simulink model "explicitaccel"  (R2021a)
settings: Solver=FixedStepAuto  StartTime=0.0  StopTime=inf  FixedStep=0.1  RelTol=1e-3
undefined symbols (not defined in the file): Angular, Linear
libraries: robotlib x20
settings Model: Creator=ivory  LastModifiedBy=sprinkle
settings SolverCC: AlgebraicLoopSolver=TrustRegion
settings OptimizationCC: EnhancedBackFolding=on  PassReuseOutputArgsAs=Individual arguments  ZeroExternalMemoryAtStartup=off  ZeroInternalMemoryAtStartup=off  MaxStackSize=64  OptimizeBlockOrder=speed  DifferentSizesBufferReuse=on  OptimizationCustomize=off  EfficientTunableParamExpr=on
settings DebuggingCC: ParameterTunabilityLossMsg=error  SFMachineParentedDataDiag=warning
settings HardwareCC: ProdBitPerPointer=32  ProdBitPerSizeT=32  ProdBitPerPtrDiffT=32  ProdLargestAtomicFloat=None  ProdIntDivRoundTo=Undefined  ProdEndianess=Unspecified  ProdWordSize=32  ProdHWDeviceType=Generic->Unspecified (assume 32-bit Generic)
settings SFSimCC: MATLABDynamicMemAlloc=off  SimTargetLang=C++
settings RTWCC: SystemTargetFile=ert.tlc  HardwareBoard=Robot Operating System (ROS)  TLCOptions="-aInlineSetEventsForThisBaseRateFcn=TLC_FALSE -aSuppressMultiTaskScheduler=TLC_FALSE  -aRateBasedStepFcn=0"  TemplateMakefile=ert_default_tmf  GenerateReport=on  Toolchain=Catkin  IncludeHyperlinkInReport=on  LaunchReport=on  TargetLang=C++  GenerateTraceInfo=on  GenerateTraceReport=on  GenerateTraceReportSl=on  GenerateTraceReportSf=on  GenerateTraceReportEml=on
settings CodeAppCC: ForceParamTrailComments=on  IgnoreCustomStorageClasses=off  OperatorAnnotations=on  SimulinkDataObjDesc=on  SFDataObjDesc=on  InsertBlockDesc=on
settings ERTTargetCC: SupportContinuousTime=on  SupportVariableSizeSignals=on

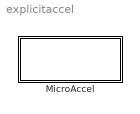
== system explicitaccel ==
  MicroAccel : Subsystem

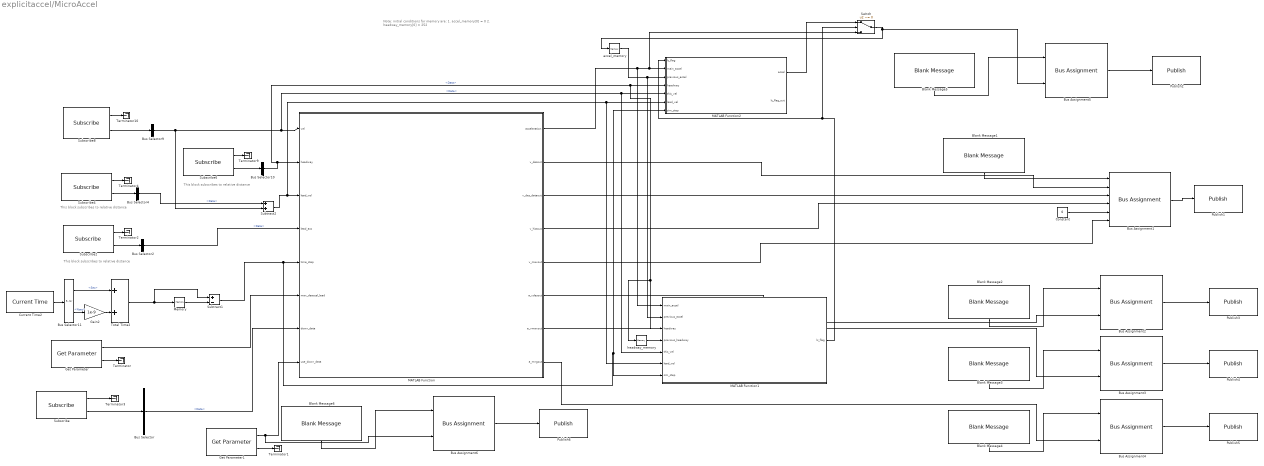
== system explicitaccel/MicroAccel ==
  note: Note: initial conditions for memory are:
      |
      | 1. accel_memory[0] = 0
      | 2. headway_memory[0] = 252
  note: This block subscribes
      | to relative distance
  note: This block subscribes
      | to relative distance
  note: This block subscribes
      | to relative distance
  Blank Message1 : robotlib/Blank Message  messageClass=Message  entityType=geometry_msgs/Twist  messageType=geometry_msgs/Twist  SampleTime=inf  legacyBusStruct=off
  Blank Message{2..5} (4 alike) : robotlib/Blank Message  messageClass=Message  entityType=std_msgs/Float64  messageType=std_msgs/Float64  SampleTime=inf  legacyBusStruct=off
  Blank Message6 : robotlib/Blank Message  messageClass=Message  entityType=std_msgs/Bool  messageType=std_msgs/Bool  SampleTime=inf  legacyBusStruct=off
  Bus Assignment1 : BusAssignment  AssignedSignals=Linear.X,Linear.Y,Linear.Z,Angular.Z,Angular.X
  Bus Assignment{2..6} (5 alike) : BusAssignment  AssignedSignals=Data
  Bus Selector{,2,4,9..10} (5 alike) : BusSelector  OutputSignals=Data
  Bus Selector11 : BusSelector  OutputSignals=Sec,Nsec
  Constant : Constant  Value=0
  Current Time2 : robotlib/Current Time  OutputFormat=bus  SampleTime=-1  ModelName=explicitaccel
      settings: SourceProductBaseCode=RR
  Gain2 : Gain  Gain=1e-9
  Get Parameter : robotlib/Get Parameter  ParameterSource=Specify your own  ParameterName=max_deaccel_lead  ParameterType=double  ParameterMaxArrayLength=16  ParameterInitialValue=-4.5  SampleTime=-1  ShowErrorCodeOutput=on  ModelName=explicitaccel  BlockId=ParamGet_explicitaccel_585
      settings: SourceProductBaseCode=RR
  Get Parameter1 : robotlib/Get Parameter  ParameterSource=Specify your own  ParameterName=use_down_data  ParameterType=boolean  ParameterMaxArrayLength=16  ParameterInitialValue=0.0  SampleTime=-1  ShowErrorCodeOutput=on  ModelName=explicitaccel  BlockId=ParamGet_explicitaccel_631
      settings: SourceProductBaseCode=RR
  MATLAB Function : MATLAB Function  TreatAsAtomicUnit=on
  MATLAB Function1 : MATLAB Function  TreatAsAtomicUnit=on
  MATLAB Function2 : MATLAB Function  TreatAsAtomicUnit=on
  Memory : Memory
  Publish1 : robotlib/Publish  topicSource=Specify your own  topic=cmd_vel  messageType=geometry_msgs/Twist  legacyBusStruct=off  messageQueueLength=1
  Publish2 : robotlib/Publish  topicSource=Specify your own  topic=cmd_accel  messageType=std_msgs/Float64  legacyBusStruct=off  messageQueueLength=1
  Publish3 : robotlib/Publish  topicSource=Specify your own  topic=a_vdesout  messageType=std_msgs/Float64  legacyBusStruct=off  messageQueueLength=1
  Publish4 : robotlib/Publish  topicSource=Specify your own  topic=a_vmaxout  messageType=std_msgs/Float64  legacyBusStruct=off  messageQueueLength=1
  Publish5 : robotlib/Publish  topicSource=Specify your own  topic=a_mngout  messageType=std_msgs/Float64  legacyBusStruct=off  messageQueueLength=1
  Publish6 : robotlib/Publish  topicSource=Specify your own  topic=downdataflag  messageType=std_msgs/Bool  legacyBusStruct=off  messageQueueLength=1
  Subscribe : robotlib/Subscribe  topicSource=Specify your own  topic=down_data  messageType=std_msgs/Float64MultiArray  SampleTime=-1  legacyBusStruct=off  messageQueueLength=1
  Subscribe2 : robotlib/Subscribe  topicSource=Specify your own  topic=lead_accel  messageType=std_msgs/Float64  SampleTime=-1  legacyBusStruct=off  messageQueueLength=1
  Subscribe4 : robotlib/Subscribe  topicSource=Specify your own  topic=rel_vel  messageType=std_msgs/Float64  SampleTime=-1  legacyBusStruct=off  messageQueueLength=1
  Subscribe6 : robotlib/Subscribe  topicSource=Specify your own  topic=lead_dist  messageType=std_msgs/Float64  SampleTime=-1  legacyBusStruct=off  messageQueueLength=1
  Subscribe8 : robotlib/Subscribe  topicSource=Specify your own  topic=vel  messageType=std_msgs/Float64  SampleTime=-1  legacyBusStruct=off  messageQueueLength=1
  Subtract1 : Sum  Inputs=+-
  Subtract2 : Sum
  Switch : Switch  Criteria=u2 ~= 0
  Terminator{,1..4,9..10} (7 alike) : Terminator
  Total Time2 : Sum
  accel_memory : Memory
  headway_memory : Memory  InitialCondition=252
  wires:
  Subscribe8/1 -> Terminator10/1
  Subscribe8/2 -> Bus Selector9/1
  Bus Selector9/1 -> MATLAB Function1/5(this_vel), MATLAB Function2/5(this_vel), MATLAB Function/1(vel), Subtract2/2  "<Data>"
  Subscribe6/1 -> Terminator9/1
  Subscribe6/2 -> Bus Selector10/1
  Bus Selector10/1 -> MATLAB Function/2(headway), headway_memory/1, MATLAB Function1/3(headway), MATLAB Function2/4(headway)  "<Data>"
  Bus Selector2/1 -> MATLAB Function/4(lead_acc)  "<Data>"
  Subscribe2/2 -> Bus Selector2/1
  Subscribe2/1 -> Terminator2/1
  Bus Selector11/1 -> Total Time2/1  "<Sec>"
  Gain2/1 -> Total Time2/2
  Bus Selector11/2 -> Gain2/1  "<Nsec>"
  Total Time2/1 -> Subtract1/1, Memory/1
  Current Time2/1 -> Bus Selector11/1
  Memory/1 -> Subtract1/2
  Subtract1/1 -> MATLAB Function2/7(sim_step), MATLAB Function1/7(sim_step), MATLAB Function/5(time_step)
  Get Parameter/2 -> Terminator/1
  Get Parameter/1 -> MATLAB Function/6(max_deaccel_lead)
  Constant/1 -> Bus Assignment1/5
  Bus Assignment1/1 -> Publish1/1
  MATLAB Function/4(v_histout) -> Bus Assignment1/4
  Blank Message1/1 -> Bus Assignment1/1
  MATLAB Function/3(v_des_dataout) -> Bus Assignment1/3
  MATLAB Function/5(v_maxout) -> Bus Assignment1/6
  MATLAB Function/7(a_vmaxout) -> Bus Assignment3/2
  MATLAB Function/2(v_desout) -> Bus Assignment1/2
  Subscribe/1 -> Terminator3/1
  Subscribe/2 -> Bus Selector/1
  Bus Selector/1 -> MATLAB Function/7(down_data)  "<Data>"
  Blank Message2/1 -> Bus Assignment2/1
  MATLAB Function/6(a_vdesout) -> Bus Assignment2/2
  Blank Message3/1 -> Bus Assignment3/1
  Blank Message4/1 -> Bus Assignment4/1
  Blank Message5/1 -> Bus Assignment5/1
  MATLAB Function/1(acceleration) -> MATLAB Function1/1(main_accel), Switch/3, MATLAB Function2/2(main_accel)
  Bus Assignment5/1 -> Publish2/1
  Bus Assignment2/1 -> Publish3/1
  Bus Assignment3/1 -> Publish4/1
  Bus Assignment4/1 -> Publish5/1
  MATLAB Function/8(a_mngout) -> Bus Assignment4/2
  Bus Selector4/1 -> Subtract2/1  "<Data>"
  Subscribe4/2 -> Bus Selector4/1
  Subscribe4/1 -> Terminator4/1
  Subtract2/1 -> MATLAB Function1/6(lead_vel), MATLAB Function2/6(lead_vel), MATLAB Function/3(lead_vel)
  Get Parameter1/2 -> Terminator1/1
  Bus Assignment6/1 -> Publish6/1
  Get Parameter1/1 -> Bus Assignment6/2, MATLAB Function/8(use_down_data)
  Blank Message6/1 -> Bus Assignment6/1
  MATLAB Function1/1(lc_flag) -> Switch/2, MATLAB Function2/1(lc_flag)
  accel_memory/1 -> MATLAB Function1/2(previous_accel), MATLAB Function2/3(previous_accel)
  headway_memory/1 -> MATLAB Function1/4(previous_headway)
  MATLAB Function2/1(accel) -> Switch/1
  Switch/1 -> Bus Assignment5/2, accel_memory/1

== matlab function explicitaccel/MicroAccel/MATLAB Function1 ==
  data: main_accel input; lc_flag output; previous_accel input; headway input; previous_headway input; this_vel input; lead_vel input; sim_step input
function lc_flag = detect_lane_change(main_accel, previous_accel, headway, previous_headway, this_vel, lead_vel, sim_step)
    lc_thresh = 3.5;
    a_comfort = 0.9 * sim_step;
    th_safe = 2;
    ttc_safe = 4.5;

    rv = lead_vel - this_vel;
    da = abs(main_accel - previous_accel);
    
    th = (this_vel > 0) * (headway / this_vel) + (this_vel <= 0) * 60;
    ttc = (rv < 0) * (-headway / rv) +  (rv >= 0) *  60;
    difference = headway - previous_headway;

    if difference <= -lc_thresh
        if da > a_comfort
            if rv >= 0 && th > th_safe
                lc_flag = -1;
                return
            elseif rv < 0 && ttc > ttc_safe
                lc_flag = -1;
                return
            end 
        end 
    elseif difference >= lc_thresh
        if da > a_comfort
            if rv >= 0 && th > th_safe
                lc_flag = 1; 
                return
            elseif rv < 0 && ttc > ttc_safe
                lc_flag = 1; 
                return
            end 
        end
    end 

    lc_flag = 0; 
end

== matlab function explicitaccel/MicroAccel/MATLAB Function ==
  data: vel input; acceleration output; headway input; lead_vel input; lead_acc input; time_step input; max_deaccel_lead input; down_data input; v_desout output; v_des_dataout output; v_histout output; v_maxout output; a_vdesout output; a_vmaxout output; a_mngout output; use_down_data input
function [acceleration, v_desout, v_des_dataout,v_histout, v_maxout, a_vdesout, a_vmaxout, a_mngout]  = Microaccel_05_22(vel, headway, lead_vel, lead_acc, time_step, max_deaccel_lead, down_data, use_down_data)
    %% Compute the desired acceleration by the Microaccel controller.
    % This model requires memory from previous time steps to properly function.
    % To achieve this, we pass the variables to be stored in memory as inputs
    % to the function, and return the updated values as outputs from it. These
    % parameters should be initialized as follows:
    % >>> time_avg_target = [];
    %
    % Parameters
    % ----------
    % vel : float
    %     the speed of the ego vehicle
    % headway : float
    %     bumper-to-bumper gap
    % lead_vel : float
    %     speed of vehicle in front
    % lead_vel : float
    %     accel of vehicle in front
    % time_step : float
    %     the average time (in seconds) in between consecutive updates
    % max_deaccel_lead : float
    %       maximal decceleration achievable by the lead vehicle
    % time_avg_target : list of float
    %     a buffer of leader speeds at previous time steps
    %
    % Returns
    % -------
    % (float, float, float, float, list of float)
    %     the desired acceleration and updated d1, d2, v_des2, and 
    %     time_avg_target terms
    %% model parameters
    max_accel = 1; %Max acceleration
    max_deaccel = -3; %Max decceleration (safety wise)
    max_deaccel_confort = -1; %Max confortable decceleration (i.e. not for safety)
    v_fast = 15;
    v_limit = 30;
    v_hist = 6;
    % to be optimized
    period = 64; 
    weight_des = 1; %parameter always equal to 1 in python, 0 means the have no gap penalty and we don't care about leader vel for v_des
    weight_hist = 0;
    weight_down = 4;
    target_time_head = 3;
    long_time_head = 5;
    h0=2.5;
    s0=2;
    k = 1; %TODO maybe decrease this parameter sometimes
    %options on the controller
    gap_variant = 1; %1 includes a gap preference for the AV, 0 only takes an average
    historical = 0; %0 assumes no past measurments on the test site, 1 uses the data from the known behavior of the traffic without AV
    
    %% Use as input
    %use_down_data = 1; %1 assures to use the downstream information, 0 is to ignore downstream data

    %% Persistent variables
    persistent previous_v_max  %the max velocity for safety in last step
    persistent previous_v_des  %the desired velocity in last step
    persistent previous_dx     %the headway in last step
    persistent time_avg_target %in order to calculate the desried velocity, time_avg_target is the column to memorize the history data
    persistent t_length        %
    average_step = 1280;%period/time_step; %the total number of memory steps
    if isempty(time_avg_target)
        t_length= 1;
        time_avg_target = zeros(1, average_step);% Data Rate = 20 Hz, To consider 64 seconds, 20*64 data points are required
        time_avg_target(average_step)= lead_vel;
    else
        time_avg_target = [time_avg_target(2:end),lead_vel];
        if(t_length < average_step)
            t_length= t_length + 1;
        end
    end
    %% Choose the desired speed based.
    % Create reference values for global target speed.
    % time_avg_target(end+1) = lead_vel
    dx = headway;
    if isempty(previous_dx)
        previous_dx = dx;
    end
    h1= target_time_head.*vel; %%%%here the target time headway is chosen as 3
    %%%%%%%%% Takes care of dowstream_data. Warning: downstream data kind
    %%%%%%%%% of overrides the headway penalization in earlier versions
    if use_down_data == 1 
        v_des_data = min(down_data); %%%%%%%%%down_data is the imported data
    else
        weight_down = 0;
        v_des_data = v_fast;
    end
    if historical == 0
        weight_hist=0;
    end
    v_des = sum(time_avg_target)/t_length; %the desired velocity from the leading vehicle
    if gap_variant == 1 %this parameter is called pen_th in python
       sum_weights = (weight_down + weight_hist + weight_des);
       v_des = (0.1.*max(0,5.*(dx-h1)./max(1, vel))^2+ v_des); %%%%%%%%%Penalise too large headway, the constants can be modified
    end
    v_des = (weight_down * v_des_data + weight_hist * v_hist + weight_des * v_des) / sum_weights; %%%%%%%%%%%%%The desired velocity based on leadign vehicle and downstream info
    %end
    
    
    if isempty(previous_v_des) 
        previous_v_des = 0;
        v_des_dot = 0;
    else
        v_des_dot = (v_des-previous_v_des)./time_step;
    end
    
    previous_v_des = v_des; %update previous_v_des
    % % Compute v_max and its derivative 
    
    v_max = sqrt(2*abs(max_deaccel)*(max(dx-s0,0)+0.5.*((lead_vel).^2)./abs(max_deaccel_lead)));
    if isempty(previous_v_max)
        previous_v_max = 0;
        v_max_dot = 0;
    elseif abs(dx-previous_dx)>time_step * 50 %Exclude the discontinuities in headway 
        v_max_dot = 0;
    else
        v_max_dot = (v_max-previous_v_max)./time_step;
    end
    
    previous_v_max = v_max; %update previous_v_max
    
    %Compute a_mng (acceleration management)
    %%%%%%%%%% Corrected
   
    a_12 = -0.5.*(vel)^2./(max(0,dx-s0)+0.5.*((lead_vel+0.001).^2)./abs(lead_acc-0.01));
    a_0 = lead_acc .* vel ./ (lead_vel + 0.001);
    if lead_acc < 0
       if a_12 > a_0   
            a_mng = a_12;
       elseif lead_vel >= vel
            a_mng = a_0;
       else    
         a_mng = lead_acc - 0.5.*(vel - lead_vel)^2 / max((dx-s0),0.001);
       end
       
    elseif lead_acc >= 0
        
        if vel >= lead_vel 
           a_mng = lead_acc - 0.5.*(vel - lead_vel)^2 / max((dx-s0),0.001);
        else
           k_2 = 1; %In python this parameter is chosen as 1 
           a_mng = min(max_accel, lead_acc + (lead_acc) * k_2 * (lead_vel - vel));
        end
    else 
        a_mng = NaN;
        "This is an error"
    end
    % %Unactivate a_mng when the vehicule is above a certain distance
     
    if dx > max(vel,lead_vel) * long_time_head %There is a change from AH.
        a_mng = max_accel;
    end
    previous_dx = dx;
    
    %% Final acceleration
    a_vdes = max(-k*(vel-v_des)+v_des_dot,-abs(max_deaccel_confort));
    a_vmax = -k*(vel-v_max)+v_max_dot;
    acceleration = min(min(a_vdes,a_vmax),a_mng);
    acceleration = min(max(acceleration, -abs(max_deaccel)), max_accel);
    
    if vel>=v_limit
        acceleration = min(0,acceleration);
    end
    
    
    %Output useful quantities
    v_desout = v_des;
    v_des_dataout = v_des_data;
    v_histout = v_hist;
    v_maxout = v_max;
    a_vdesout = a_vdes;
    a_vmaxout = a_vmax;
    a_mngout = a_mng;
    end

== matlab function explicitaccel/MicroAccel/MATLAB Function2 ==
  data: lc_flag input; accel output; main_accel input; previous_accel input; headway input; this_vel input; lead_vel input; sim_step input; lc_flag_out output
function [accel, lc_flag_out] = get_lc_recovery_accel(lc_flag, ...
                               main_accel, previous_accel, ...
                               headway, this_vel, lead_vel, sim_step)
    h_star = 1.32;
    rv_star_positive = 1;
    rv_star_negative = 10.34/headway; 
    epsilon = 0.3 * sim_step;
    f_h = 0.75;
    f_rv = 0.25;
    
    th = (this_vel > 0) * (headway / this_vel) + (this_vel <= 0) * 60;
    rv = lead_vel - this_vel; 
    rv_star = rv_star_positive * (rv >= 0) + rv_star_negative * (rv < 0);
    
    alpha = f_h * tanh(h_star * th) + f_rv * (0.5 * tanh(rv_star * rv) + 0.5);
    recovery_accel = alpha * previous_accel + (1 - alpha) * main_accel;
    
    if abs(recovery_accel - main_accel) < epsilon
        accel = main_accel; 
        lc_flag_out = 0; 
    else
        accel = recovery_accel; 
        lc_flag_out = lc_flag; 
    end
end
